simulink model "UART"  (R2025a)
settings: Solver=FixedStepAuto  StartTime=0.0  StopTime=10  FixedStep=1e-6  RelTol=1e-3
undefined symbols (not defined in the file): Bit_1, Bit_2, Bit_3, Bit_4, Bit_5, Bit_6, Bit_7, Bit_8
libraries: simulink_extras x158, fl_lib x17, nesl_utility x8, simulink x7
(part 3 of 6)

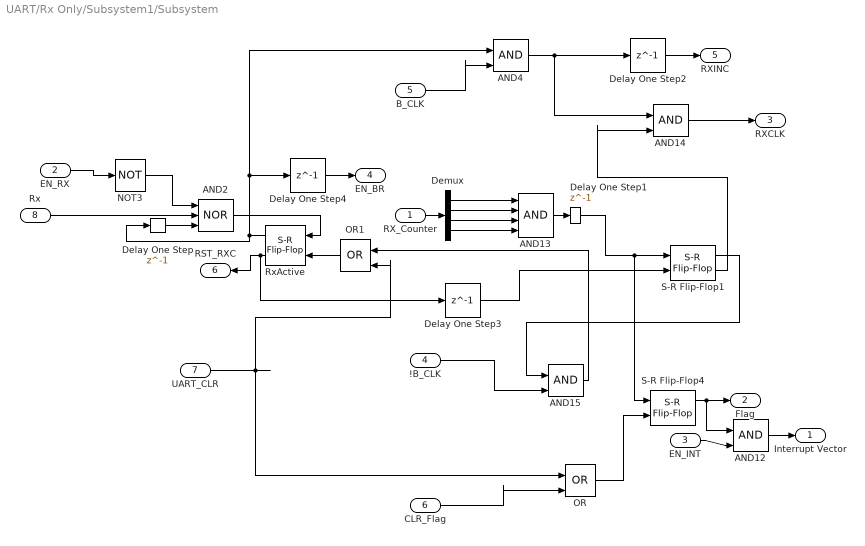
== system UART/Rx Only/Subsystem1/Subsystem ==
  RX_Counter : Inport
  EN_RX : Inport  Port=2
  EN_INT : Inport  Port=3
  !B_CLK : Inport  Port=4
  B_CLK : Inport  Port=5
  CLR_Flag : Inport  Port=6
  UART_CLR : Inport  Port=7
  Rx : Inport  Port=8
  AND{4,12,14..15} (4 alike) : Logic  IconShape=distinctive  AllPortsSameDT=off  OutDataTypeStr=boolean
  AND13 : Logic  Inputs=4  IconShape=distinctive  AllPortsSameDT=off  OutDataTypeStr=boolean
  AND2 : Logic  Operator=NOR  Inputs=3  IconShape=distinctive  AllPortsSameDT=off  OutDataTypeStr=boolean
  Delay One Step{,1..4} (5 alike) : Delay  DelayLength=1
  Demux : Demux
  NOT3 : Logic  Operator=NOT  IconShape=distinctive  AllPortsSameDT=off  OutDataTypeStr=boolean
  OR : Logic  Operator=OR  IconShape=distinctive  AllPortsSameDT=off  OutDataTypeStr=boolean
  OR1 : Logic  Operator=OR  IconShape=distinctive  AllPortsSameDT=off  OutDataTypeStr=boolean
  RxActive : simulink_extras/Flip Flops/S-R Flip-Flop  initial_condition=0
  S-R Flip-Flop1 : simulink_extras/Flip Flops/S-R Flip-Flop  initial_condition=0
  S-R Flip-Flop4 : simulink_extras/Flip Flops/S-R Flip-Flop  initial_condition=0
  Interrupt Vector : Outport
  Flag : Outport  Port=2
  RXCLK : Outport  Port=3
  EN_BR : Outport  Port=4
  RXINC : Outport  Port=5
  RST_RXC : Outport  Port=6
  wires:
  UART_CLR/1 -> OR/1, OR1/2
  !B_CLK/1 -> AND15/2
  Rx/1 -> AND2/2
  EN_RX/1 -> NOT3/1
  AND2/1 -> RxActive/1
  EN_INT/1 -> AND12/2
  S-R Flip-Flop4/1 -> AND12/1, Flag/1
  AND12/1 -> Interrupt Vector/1
  CLR_Flag/1 -> OR/2
  RxActive/2 -> Delay One Step3/1, RST_RXC/1
  Demux/1 -> AND13/1
  Demux/2 -> AND13/2
  B_CLK/1 -> AND4/2
  AND4/1 -> Delay One Step2/1, AND14/1
  RX_Counter/1 -> Demux/1
  Delay One Step1/1 -> S-R Flip-Flop4/1, S-R Flip-Flop1/1
  AND15/1 -> OR1/1
  RxActive/1 -> Delay One Step/1, Delay One Step4/1, AND4/1
  Demux/3 -> AND13/3
  Demux/4 -> AND13/4
  Delay One Step2/1 -> RXINC/1
  AND14/1 -> RXCLK/1
  S-R Flip-Flop1/2 -> AND14/2
  OR1/1 -> RxActive/2
  NOT3/1 -> AND2/1
  Delay One Step/1 -> AND2/3
  AND13/1 -> Delay One Step1/1
  OR/1 -> S-R Flip-Flop4/2
  S-R Flip-Flop1/1 -> AND15/1
  Delay One Step3/1 -> S-R Flip-Flop1/2
  Delay One Step4/1 -> EN_BR/1

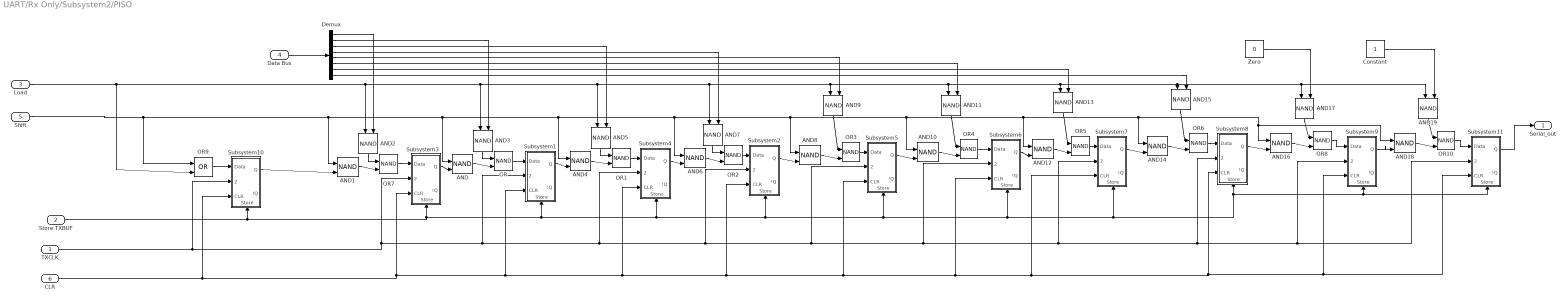
== system UART/Rx Only/Subsystem2/PISO ==
  "TXCLK " : Inport
  Store TXBUF : Inport  Port=2
  Load : Inport  Port=3
  Data Bus : Inport  Port=4
  Shift : Inport  Port=5
  "CLR " : Inport  Port=6
  AND{,1..19} (20 alike) : Logic  Operator=NAND  IconShape=distinctive  AllPortsSameDT=off  OutDataTypeStr=boolean
  Constant : Constant
  Demux : Demux  Outputs=8
  OR{,1..8,10} (10 alike) : Logic  Operator=NAND  IconShape=distinctive  AllPortsSameDT=off  OutDataTypeStr=boolean
  OR9 : Logic  Operator=OR  IconShape=distinctive  AllPortsSameDT=off  OutDataTypeStr=boolean
  Subsystem1 : Subsystem
      settings: PortSchema="{\"entries\":[{\"content\":{\"sides\":[{\"content\":{\"connectorIds\":[\"In1\",\"In2\",\"In3\"]},\"type\":\"ConnectorPlacement.EquallySpacedRectSide\",\"uuid\":\"7f3c85a8-435a-48c3-b59c-f5d5714c847e\"},{\"content\":{\"connectorIds\":[\"Out1\",\"Out2\"],\"side\":\"RIGHT\"},\"type\":\"ConnectorPlacement.EquallySpacedRectSide\",\"uuid\":\"17207f13-8340-45d6-91b4-1610668ce323\"},{\"content\":{\"side\":\"TOP\"},\"type\":\"ConnectorPlacement.EquallySpacedRectSide\",\"uuid\":\"04d61695-a4c9-4852-a4b1-2cdbdbfa921f\"},{\"content\":{\"connectorIds\":[\"In4\"],\"side\":\"BOTTOM\"},\"type\":\"ConnectorPlacement.EquallySpacedRectSide\",\"uuid\":\"a1770489-59eb-478b-9b54-00148a18765c\"}]},\"type\":\"ConnectorPlacement.EquallySpacedConnector\",\"uuid\":\"06dc9f9c-9f45-42f3-b967-f8303bc685fc\"}],\"packageUris\":[\"http://schema.mathworks.com/mf0/Connector/R2020b\"],\"version\":\"1.0\"}"
  Subsystem10 : Subsystem
      settings: PortSchema="{\"entries\":[{\"content\":{\"sides\":[{\"content\":{\"connectorIds\":[\"In1\",\"In2\",\"In3\"]},\"type\":\"ConnectorPlacement.EquallySpacedRectSide\",\"uuid\":\"7f3c85a8-435a-48c3-b59c-f5d5714c847e\"},{\"content\":{\"connectorIds\":[\"Out1\",\"Out2\"],\"side\":\"RIGHT\"},\"type\":\"ConnectorPlacement.EquallySpacedRectSide\",\"uuid\":\"17207f13-8340-45d6-91b4-1610668ce323\"},{\"content\":{\"side\":\"TOP\"},\"type\":\"ConnectorPlacement.EquallySpacedRectSide\",\"uuid\":\"04d61695-a4c9-4852-a4b1-2cdbdbfa921f\"},{\"content\":{\"connectorIds\":[\"In4\"],\"side\":\"BOTTOM\"},\"type\":\"ConnectorPlacement.EquallySpacedRectSide\",\"uuid\":\"a1770489-59eb-478b-9b54-00148a18765c\"}]},\"type\":\"ConnectorPlacement.EquallySpacedConnector\",\"uuid\":\"06dc9f9c-9f45-42f3-b967-f8303bc685fc\"}],\"packageUris\":[\"http://schema.mathworks.com/mf0/Connector/R2020b\"],\"version\":\"1.0\"}"
  Subsystem11 : Subsystem
      settings: PortSchema="{\"entries\":[{\"content\":{\"sides\":[{\"content\":{\"connectorIds\":[\"In1\",\"In2\",\"In3\"]},\"type\":\"ConnectorPlacement.EquallySpacedRectSide\",\"uuid\":\"7f3c85a8-435a-48c3-b59c-f5d5714c847e\"},{\"content\":{\"connectorIds\":[\"Out1\",\"Out2\"],\"side\":\"RIGHT\"},\"type\":\"ConnectorPlacement.EquallySpacedRectSide\",\"uuid\":\"17207f13-8340-45d6-91b4-1610668ce323\"},{\"content\":{\"side\":\"TOP\"},\"type\":\"ConnectorPlacement.EquallySpacedRectSide\",\"uuid\":\"04d61695-a4c9-4852-a4b1-2cdbdbfa921f\"},{\"content\":{\"connectorIds\":[\"In4\"],\"side\":\"BOTTOM\"},\"type\":\"ConnectorPlacement.EquallySpacedRectSide\",\"uuid\":\"a1770489-59eb-478b-9b54-00148a18765c\"}]},\"type\":\"ConnectorPlacement.EquallySpacedConnector\",\"uuid\":\"06dc9f9c-9f45-42f3-b967-f8303bc685fc\"}],\"packageUris\":[\"http://schema.mathworks.com/mf0/Connector/R2020b\"],\"version\":\"1.0\"}"
  Subsystem2 : Subsystem
      settings: PortSchema="{\"entries\":[{\"content\":{\"sides\":[{\"content\":{\"connectorIds\":[\"In1\",\"In2\",\"In3\"]},\"type\":\"ConnectorPlacement.EquallySpacedRectSide\",\"uuid\":\"7f3c85a8-435a-48c3-b59c-f5d5714c847e\"},{\"content\":{\"connectorIds\":[\"Out1\",\"Out2\"],\"side\":\"RIGHT\"},\"type\":\"ConnectorPlacement.EquallySpacedRectSide\",\"uuid\":\"17207f13-8340-45d6-91b4-1610668ce323\"},{\"content\":{\"side\":\"TOP\"},\"type\":\"ConnectorPlacement.EquallySpacedRectSide\",\"uuid\":\"04d61695-a4c9-4852-a4b1-2cdbdbfa921f\"},{\"content\":{\"connectorIds\":[\"In4\"],\"side\":\"BOTTOM\"},\"type\":\"ConnectorPlacement.EquallySpacedRectSide\",\"uuid\":\"a1770489-59eb-478b-9b54-00148a18765c\"}]},\"type\":\"ConnectorPlacement.EquallySpacedConnector\",\"uuid\":\"06dc9f9c-9f45-42f3-b967-f8303bc685fc\"}],\"packageUris\":[\"http://schema.mathworks.com/mf0/Connector/R2020b\"],\"version\":\"1.0\"}"
  Subsystem3 : Subsystem
      settings: PortSchema="{\"entries\":[{\"content\":{\"sides\":[{\"content\":{\"connectorIds\":[\"In1\",\"In2\",\"In3\"]},\"type\":\"ConnectorPlacement.EquallySpacedRectSide\",\"uuid\":\"7f3c85a8-435a-48c3-b59c-f5d5714c847e\"},{\"content\":{\"connectorIds\":[\"Out1\",\"Out2\"],\"side\":\"RIGHT\"},\"type\":\"ConnectorPlacement.EquallySpacedRectSide\",\"uuid\":\"17207f13-8340-45d6-91b4-1610668ce323\"},{\"content\":{\"side\":\"TOP\"},\"type\":\"ConnectorPlacement.EquallySpacedRectSide\",\"uuid\":\"04d61695-a4c9-4852-a4b1-2cdbdbfa921f\"},{\"content\":{\"connectorIds\":[\"In4\"],\"side\":\"BOTTOM\"},\"type\":\"ConnectorPlacement.EquallySpacedRectSide\",\"uuid\":\"a1770489-59eb-478b-9b54-00148a18765c\"}]},\"type\":\"ConnectorPlacement.EquallySpacedConnector\",\"uuid\":\"06dc9f9c-9f45-42f3-b967-f8303bc685fc\"}],\"packageUris\":[\"http://schema.mathworks.com/mf0/Connector/R2020b\"],\"version\":\"1.0\"}"
  Subsystem4 : Subsystem
      settings: PortSchema="{\"entries\":[{\"content\":{\"sides\":[{\"content\":{\"connectorIds\":[\"In1\",\"In2\",\"In3\"]},\"type\":\"ConnectorPlacement.EquallySpacedRectSide\",\"uuid\":\"7f3c85a8-435a-48c3-b59c-f5d5714c847e\"},{\"content\":{\"connectorIds\":[\"Out1\",\"Out2\"],\"side\":\"RIGHT\"},\"type\":\"ConnectorPlacement.EquallySpacedRectSide\",\"uuid\":\"17207f13-8340-45d6-91b4-1610668ce323\"},{\"content\":{\"side\":\"TOP\"},\"type\":\"ConnectorPlacement.EquallySpacedRectSide\",\"uuid\":\"04d61695-a4c9-4852-a4b1-2cdbdbfa921f\"},{\"content\":{\"connectorIds\":[\"In4\"],\"side\":\"BOTTOM\"},\"type\":\"ConnectorPlacement.EquallySpacedRectSide\",\"uuid\":\"a1770489-59eb-478b-9b54-00148a18765c\"}]},\"type\":\"ConnectorPlacement.EquallySpacedConnector\",\"uuid\":\"06dc9f9c-9f45-42f3-b967-f8303bc685fc\"}],\"packageUris\":[\"http://schema.mathworks.com/mf0/Connector/R2020b\"],\"version\":\"1.0\"}"
  Subsystem5 : Subsystem
      settings: PortSchema="{\"entries\":[{\"content\":{\"sides\":[{\"content\":{\"connectorIds\":[\"In1\",\"In2\",\"In3\"]},\"type\":\"ConnectorPlacement.EquallySpacedRectSide\",\"uuid\":\"7f3c85a8-435a-48c3-b59c-f5d5714c847e\"},{\"content\":{\"connectorIds\":[\"Out1\",\"Out2\"],\"side\":\"RIGHT\"},\"type\":\"ConnectorPlacement.EquallySpacedRectSide\",\"uuid\":\"17207f13-8340-45d6-91b4-1610668ce323\"},{\"content\":{\"side\":\"TOP\"},\"type\":\"ConnectorPlacement.EquallySpacedRectSide\",\"uuid\":\"04d61695-a4c9-4852-a4b1-2cdbdbfa921f\"},{\"content\":{\"connectorIds\":[\"In4\"],\"side\":\"BOTTOM\"},\"type\":\"ConnectorPlacement.EquallySpacedRectSide\",\"uuid\":\"a1770489-59eb-478b-9b54-00148a18765c\"}]},\"type\":\"ConnectorPlacement.EquallySpacedConnector\",\"uuid\":\"06dc9f9c-9f45-42f3-b967-f8303bc685fc\"}],\"packageUris\":[\"http://schema.mathworks.com/mf0/Connector/R2020b\"],\"version\":\"1.0\"}"
  Subsystem6 : Subsystem
      settings: PortSchema="{\"entries\":[{\"content\":{\"sides\":[{\"content\":{\"connectorIds\":[\"In1\",\"In2\",\"In3\"]},\"type\":\"ConnectorPlacement.EquallySpacedRectSide\",\"uuid\":\"7f3c85a8-435a-48c3-b59c-f5d5714c847e\"},{\"content\":{\"connectorIds\":[\"Out1\",\"Out2\"],\"side\":\"RIGHT\"},\"type\":\"ConnectorPlacement.EquallySpacedRectSide\",\"uuid\":\"17207f13-8340-45d6-91b4-1610668ce323\"},{\"content\":{\"side\":\"TOP\"},\"type\":\"ConnectorPlacement.EquallySpacedRectSide\",\"uuid\":\"04d61695-a4c9-4852-a4b1-2cdbdbfa921f\"},{\"content\":{\"connectorIds\":[\"In4\"],\"side\":\"BOTTOM\"},\"type\":\"ConnectorPlacement.EquallySpacedRectSide\",\"uuid\":\"a1770489-59eb-478b-9b54-00148a18765c\"}]},\"type\":\"ConnectorPlacement.EquallySpacedConnector\",\"uuid\":\"06dc9f9c-9f45-42f3-b967-f8303bc685fc\"}],\"packageUris\":[\"http://schema.mathworks.com/mf0/Connector/R2020b\"],\"version\":\"1.0\"}"
  Subsystem7 : Subsystem
      settings: PortSchema="{\"entries\":[{\"content\":{\"sides\":[{\"content\":{\"connectorIds\":[\"In1\",\"In2\",\"In3\"]},\"type\":\"ConnectorPlacement.EquallySpacedRectSide\",\"uuid\":\"7f3c85a8-435a-48c3-b59c-f5d5714c847e\"},{\"content\":{\"connectorIds\":[\"Out1\",\"Out2\"],\"side\":\"RIGHT\"},\"type\":\"ConnectorPlacement.EquallySpacedRectSide\",\"uuid\":\"17207f13-8340-45d6-91b4-1610668ce323\"},{\"content\":{\"side\":\"TOP\"},\"type\":\"ConnectorPlacement.EquallySpacedRectSide\",\"uuid\":\"04d61695-a4c9-4852-a4b1-2cdbdbfa921f\"},{\"content\":{\"connectorIds\":[\"In4\"],\"side\":\"BOTTOM\"},\"type\":\"ConnectorPlacement.EquallySpacedRectSide\",\"uuid\":\"a1770489-59eb-478b-9b54-00148a18765c\"}]},\"type\":\"ConnectorPlacement.EquallySpacedConnector\",\"uuid\":\"06dc9f9c-9f45-42f3-b967-f8303bc685fc\"}],\"packageUris\":[\"http://schema.mathworks.com/mf0/Connector/R2020b\"],\"version\":\"1.0\"}"
  Subsystem8 : Subsystem
      settings: PortSchema="{\"entries\":[{\"content\":{\"sides\":[{\"content\":{\"connectorIds\":[\"In1\",\"In2\",\"In3\"]},\"type\":\"ConnectorPlacement.EquallySpacedRectSide\",\"uuid\":\"7f3c85a8-435a-48c3-b59c-f5d5714c847e\"},{\"content\":{\"connectorIds\":[\"Out1\",\"Out2\"],\"side\":\"RIGHT\"},\"type\":\"ConnectorPlacement.EquallySpacedRectSide\",\"uuid\":\"17207f13-8340-45d6-91b4-1610668ce323\"},{\"content\":{\"side\":\"TOP\"},\"type\":\"ConnectorPlacement.EquallySpacedRectSide\",\"uuid\":\"04d61695-a4c9-4852-a4b1-2cdbdbfa921f\"},{\"content\":{\"connectorIds\":[\"In4\"],\"side\":\"BOTTOM\"},\"type\":\"ConnectorPlacement.EquallySpacedRectSide\",\"uuid\":\"a1770489-59eb-478b-9b54-00148a18765c\"}]},\"type\":\"ConnectorPlacement.EquallySpacedConnector\",\"uuid\":\"06dc9f9c-9f45-42f3-b967-f8303bc685fc\"}],\"packageUris\":[\"http://schema.mathworks.com/mf0/Connector/R2020b\"],\"version\":\"1.0\"}"
  Subsystem9 : Subsystem
      settings: PortSchema="{\"entries\":[{\"content\":{\"sides\":[{\"content\":{\"connectorIds\":[\"In1\",\"In2\",\"In3\"]},\"type\":\"ConnectorPlacement.EquallySpacedRectSide\",\"uuid\":\"7f3c85a8-435a-48c3-b59c-f5d5714c847e\"},{\"content\":{\"connectorIds\":[\"Out1\",\"Out2\"],\"side\":\"RIGHT\"},\"type\":\"ConnectorPlacement.EquallySpacedRectSide\",\"uuid\":\"17207f13-8340-45d6-91b4-1610668ce323\"},{\"content\":{\"side\":\"TOP\"},\"type\":\"ConnectorPlacement.EquallySpacedRectSide\",\"uuid\":\"04d61695-a4c9-4852-a4b1-2cdbdbfa921f\"},{\"content\":{\"connectorIds\":[\"In4\"],\"side\":\"BOTTOM\"},\"type\":\"ConnectorPlacement.EquallySpacedRectSide\",\"uuid\":\"a1770489-59eb-478b-9b54-00148a18765c\"}]},\"type\":\"ConnectorPlacement.EquallySpacedConnector\",\"uuid\":\"06dc9f9c-9f45-42f3-b967-f8303bc685fc\"}],\"packageUris\":[\"http://schema.mathworks.com/mf0/Connector/R2020b\"],\"version\":\"1.0\"}"
  Zero : Constant  Value=0  OutDataTypeStr=Inherit: Inherit via back propagation
  Serial_out : Outport
  wires:
  AND12/1 -> OR5/2
  AND14/1 -> OR6/2
  AND13/1 -> OR5/1
  OR6/1 -> Subsystem8/1(Data)
  AND6/1 -> OR2/2
  AND7/1 -> OR2/1
  Subsystem4/1(Q) -> AND6/2
  OR2/1 -> Subsystem2/1(Data)
  Subsystem2/1(Q) -> AND8/2
  AND15/1 -> OR6/1
  AND8/1 -> OR3/2
  AND3/1 -> OR/1
  OR5/1 -> Subsystem7/1(Data)
  Subsystem7/1(Q) -> AND14/2
  AND11/1 -> OR4/1
  AND9/1 -> OR3/1
  Subsystem6/1(Q) -> AND12/2
  OR3/1 -> Subsystem5/1(Data)
  OR4/1 -> Subsystem6/1(Data)
  OR1/1 -> Subsystem4/1(Data)
  AND5/1 -> OR1/1
  AND/1 -> OR/2
  AND4/1 -> OR1/2
  Subsystem1/1(Q) -> AND4/2
  Subsystem3/1(Q) -> AND/2
  OR/1 -> Subsystem1/1(Data)
  OR7/1 -> Subsystem3/1(Data)
  Subsystem5/1(Q) -> AND10/2
  AND10/1 -> OR4/2
  Data Bus/1 -> Demux/1
  AND2/1 -> OR7/1
  AND1/1 -> OR7/2
  Subsystem8/1(Q) -> AND16/2
  Subsystem10/1(Q) -> AND1/2
  Demux/1 -> AND2/2
  Demux/2 -> AND3/2
  Demux/3 -> AND5/2
  Demux/4 -> AND7/2
  Demux/5 -> AND9/2
  Demux/6 -> AND11/2
  Demux/7 -> AND13/2
  Demux/8 -> AND15/2
  AND16/1 -> OR8/2
  OR8/1 -> Subsystem9/1(Data)
  AND17/1 -> OR8/1
  Zero/1 -> AND17/2
  OR9/1 -> Subsystem10/1(Data)
  Subsystem11/1(Q) -> Serial_out/1
  Load/1 -> OR9/2, AND2/1, AND3/1, AND5/1, AND7/1, AND9/1, AND11/1, AND13/1, AND19/1, AND17/1, AND15/1
  OR10/1 -> Subsystem11/1(Data)
  "TXCLK "/1 -> Subsystem10/2(Clock), Subsystem3/2(Clock), Subsystem1/2(Clock), Subsystem4/2(Clock), Subsystem2/2(Clock), Subsystem5/2(Clock), Subsystem6/2(Clock), Subsystem11/2(Clock), Subsystem9/2(Clock), Subsystem8/2(Clock), Subsystem7/2(Clock)
  Subsystem9/1(Q) -> AND18/2
  AND19/1 -> OR10/1
  AND18/1 -> OR10/2
  Store TXBUF/1 -> Subsystem10/4(Store), Subsystem3/4(Store), Subsystem1/4(Store), Subsystem4/4(Store), Subsystem2/4(Store), Subsystem5/4(Store), Subsystem6/4(Store), Subsystem11/4(Store), Subsystem9/4(Store), Subsystem8/4(Store), Subsystem7/4(Store)
  Constant/1 -> AND19/2
  "CLR "/1 -> Subsystem10/3(CLR), Subsystem3/3(CLR), Subsystem1/3(CLR), Subsystem4/3(CLR), Subsystem2/3(CLR), Subsystem5/3(CLR), Subsystem6/3(CLR), Subsystem11/3(CLR), Subsystem9/3(CLR), Subsystem8/3(CLR), Subsystem7/3(CLR)
  Shift/1 -> OR9/1, AND1/1, AND6/1, AND10/1, AND12/1, AND18/1, AND16/1, AND14/1, AND8/1, AND4/1, AND/1

== system UART/Rx Only/Subsystem2/RX Counter1 ==
  BC_Reset : Inport
  INC : Inport  Port=2
  Constant : Constant
  D Flip-Flop{5..7,11} (4 alike) : simulink_extras/Flip Flops/D Flip-Flop
  Delay One Step : Delay  DelayLength=1
  Demux : Demux
  Half Adder : Subsystem
      settings: PortSchema="{\"entries\":[{\"content\":{\"sides\":[{\"content\":{\"connectorIds\":[\"In1\"]},\"type\":\"ConnectorPlacement.EquallySpacedRectSide\",\"uuid\":\"d3a7e232-15f2-47a9-a065-9480c81dc57e\"},{\"content\":{\"connectorIds\":[\"Out1\"],\"side\":\"RIGHT\"},\"type\":\"ConnectorPlacement.EquallySpacedRectSide\",\"uuid\":\"e118f150-fee7-4aeb-941e-53c3f02c6791\"},{\"content\":{\"connectorIds\":[\"Out2\"],\"side\":\"TOP\"},\"type\":\"ConnectorPlacement.EquallySpacedRectSide\",\"uuid\":\"6d9038ab-faad-455b-a9c5-8fe0bbf34e51\"},{\"content\":{\"connectorIds\":[\"In2\"],\"side\":\"BOTTOM\"},\"type\":\"ConnectorPlacement.EquallySpacedRectSide\",\"uuid\":\"d09c8d4f-08f3-4c52-88a6-8c6db517fc7a\"}]},\"type\":\"ConnectorPlacement.EquallySpacedConnector\",\"uuid\":\"5bc947ce-f1cd-4957-9186-40c14c78de7d\"}],\"packageUris\":[\"http://schema.mathworks.com/mf0/Connector/R2020b\"],\"version\":\"1.0\"}"
  Half Adder1 : Subsystem
      settings: PortSchema="{\"entries\":[{\"content\":{\"sides\":[{\"content\":{\"connectorIds\":[\"In1\"]},\"type\":\"ConnectorPlacement.EquallySpacedRectSide\",\"uuid\":\"d3a7e232-15f2-47a9-a065-9480c81dc57e\"},{\"content\":{\"connectorIds\":[\"Out1\"],\"side\":\"RIGHT\"},\"type\":\"ConnectorPlacement.EquallySpacedRectSide\",\"uuid\":\"e118f150-fee7-4aeb-941e-53c3f02c6791\"},{\"content\":{\"connectorIds\":[\"Out2\"],\"side\":\"TOP\"},\"type\":\"ConnectorPlacement.EquallySpacedRectSide\",\"uuid\":\"6d9038ab-faad-455b-a9c5-8fe0bbf34e51\"},{\"content\":{\"connectorIds\":[\"In2\"],\"side\":\"BOTTOM\"},\"type\":\"ConnectorPlacement.EquallySpacedRectSide\",\"uuid\":\"d09c8d4f-08f3-4c52-88a6-8c6db517fc7a\"}]},\"type\":\"ConnectorPlacement.EquallySpacedConnector\",\"uuid\":\"5bc947ce-f1cd-4957-9186-40c14c78de7d\"}],\"packageUris\":[\"http://schema.mathworks.com/mf0/Connector/R2020b\"],\"version\":\"1.0\"}"
  Half Adder2 : Subsystem
      settings: PortSchema="{\"entries\":[{\"content\":{\"sides\":[{\"content\":{\"connectorIds\":[\"In1\"]},\"type\":\"ConnectorPlacement.EquallySpacedRectSide\",\"uuid\":\"d3a7e232-15f2-47a9-a065-9480c81dc57e\"},{\"content\":{\"connectorIds\":[\"Out1\"],\"side\":\"RIGHT\"},\"type\":\"ConnectorPlacement.EquallySpacedRectSide\",\"uuid\":\"e118f150-fee7-4aeb-941e-53c3f02c6791\"},{\"content\":{\"connectorIds\":[\"Out2\"],\"side\":\"TOP\"},\"type\":\"ConnectorPlacement.EquallySpacedRectSide\",\"uuid\":\"6d9038ab-faad-455b-a9c5-8fe0bbf34e51\"},{\"content\":{\"connectorIds\":[\"In2\"],\"side\":\"BOTTOM\"},\"type\":\"ConnectorPlacement.EquallySpacedRectSide\",\"uuid\":\"d09c8d4f-08f3-4c52-88a6-8c6db517fc7a\"}]},\"type\":\"ConnectorPlacement.EquallySpacedConnector\",\"uuid\":\"5bc947ce-f1cd-4957-9186-40c14c78de7d\"}],\"packageUris\":[\"http://schema.mathworks.com/mf0/Connector/R2020b\"],\"version\":\"1.0\"}"
  Half Adder7 : Subsystem
      settings: PortSchema="{\"entries\":[{\"content\":{\"sides\":[{\"content\":{\"connectorIds\":[\"In1\"]},\"type\":\"ConnectorPlacement.EquallySpacedRectSide\",\"uuid\":\"d3a7e232-15f2-47a9-a065-9480c81dc57e\"},{\"content\":{\"connectorIds\":[\"Out1\"],\"side\":\"RIGHT\"},\"type\":\"ConnectorPlacement.EquallySpacedRectSide\",\"uuid\":\"e118f150-fee7-4aeb-941e-53c3f02c6791\"},{\"content\":{\"connectorIds\":[\"Out2\"],\"side\":\"TOP\"},\"type\":\"ConnectorPlacement.EquallySpacedRectSide\",\"uuid\":\"6d9038ab-faad-455b-a9c5-8fe0bbf34e51\"},{\"content\":{\"connectorIds\":[\"In2\"],\"side\":\"BOTTOM\"},\"type\":\"ConnectorPlacement.EquallySpacedRectSide\",\"uuid\":\"d09c8d4f-08f3-4c52-88a6-8c6db517fc7a\"}]},\"type\":\"ConnectorPlacement.EquallySpacedConnector\",\"uuid\":\"5bc947ce-f1cd-4957-9186-40c14c78de7d\"}],\"packageUris\":[\"http://schema.mathworks.com/mf0/Connector/R2020b\"],\"version\":\"1.0\"}"
  Mux1 : Mux
  NOT : Logic  Operator=NOT  IconShape=distinctive  AllPortsSameDT=off  OutDataTypeStr=boolean
  C4 : Outport
  !C3 : Outport  Port=2
  C2 : Outport  Port=3
  C1 : Outport  Port=4
  wires:
  Mux1/1 -> Delay One Step/1
  BC_Reset/1 -> NOT/1
  Delay One Step/1 -> Demux/1
  Demux/4 -> D Flip-Flop7/1
  Demux/3 -> D Flip-Flop5/1
  Demux/2 -> D Flip-Flop6/1
  Demux/1 -> D Flip-Flop11/1
  INC/1 -> D Flip-Flop11/2, D Flip-Flop6/2, D Flip-Flop5/2, D Flip-Flop7/2
  Constant/1 -> Half Adder7/2("B ")
  Half Adder/2(Carry) -> Half Adder1/2("B ")
  Half Adder1/1(Sum) -> Mux1/2
  Half Adder/1(Sum) -> Mux1/3
  Half Adder2/1(Sum) -> Mux1/1
  Half Adder1/2(Carry) -> Half Adder2/2("B ")
  Half Adder7/1(Sum) -> Mux1/4
  Half Adder7/2(Carry) -> Half Adder/2("B ")
  D Flip-Flop11/1 -> C4/1, Half Adder2/1(A)  "D1"
  D Flip-Flop6/1 -> Half Adder1/1(A)  "D3"
  D Flip-Flop5/1 -> C2/1, Half Adder/1(A)  "D4"
  D Flip-Flop7/1 -> C1/1, Half Adder7/1(A)  "D2"
  NOT/1 -> D Flip-Flop11/3, D Flip-Flop6/3, D Flip-Flop5/3, D Flip-Flop7/3
  D Flip-Flop6/2 -> !C3/1

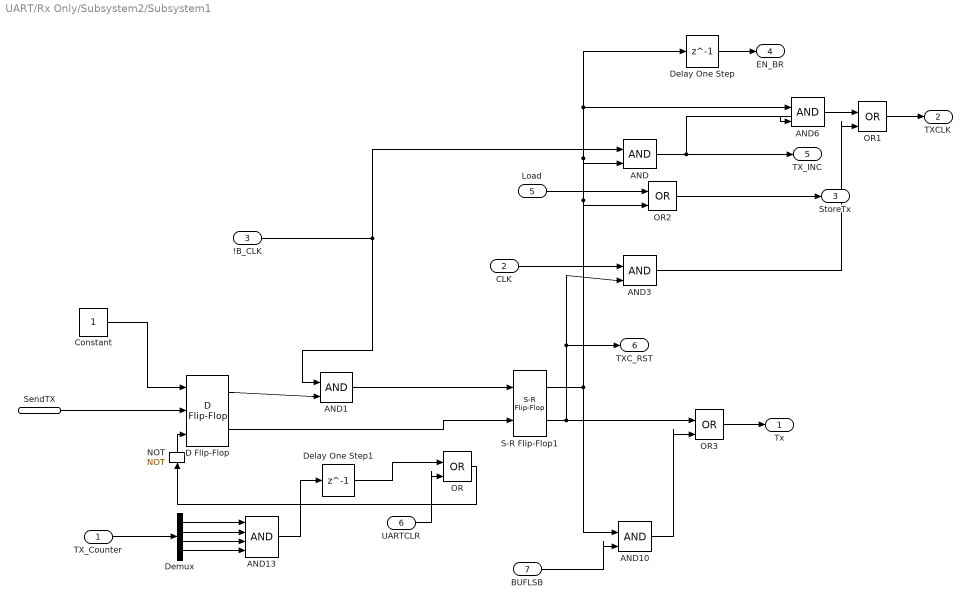
== system UART/Rx Only/Subsystem2/Subsystem1 ==
  TX_Counter : Inport
  CLK : Inport  Port=2
  !B_CLK : Inport  Port=3
  SendTX : Inport  Port=4
  Load : Inport  Port=5
  UARTCLR : Inport  Port=6
  BUFLSB : Inport  Port=7
  AND{,1,3,6,10} (5 alike) : Logic  IconShape=distinctive  AllPortsSameDT=off  OutDataTypeStr=boolean
  AND13 : Logic  Inputs=4  IconShape=distinctive  AllPortsSameDT=off  OutDataTypeStr=boolean
  Constant : Constant  OutDataTypeStr=boolean
  D Flip-Flop : simulink_extras/Flip Flops/D Flip-Flop
  Delay One Step : Delay  DelayLength=1
  Delay One Step1 : Delay  DelayLength=1  SampleTime=1e-5
  Demux : Demux
  NOT : Logic  Operator=NOT  IconShape=distinctive  AllPortsSameDT=off  OutDataTypeStr=boolean
  OR{,1..3} (4 alike) : Logic  Operator=OR  IconShape=distinctive  AllPortsSameDT=off  OutDataTypeStr=boolean
  S-R Flip-Flop1 : simulink_extras/Flip Flops/S-R Flip-Flop  initial_condition=0
  Tx : Outport
  TXCLK : Outport  Port=2
  StoreTx : Outport  Port=3
  EN_BR : Outport  Port=4
  TX_INC : Outport  Port=5
  TXC_RST : Outport  Port=6
  wires:
  OR2/1 -> StoreTx/1
  AND3/1 -> OR1/2
  S-R Flip-Flop1/2 -> AND3/2, TXC_RST/1, OR3/1
  CLK/1 -> AND3/1
  OR1/1 -> TXCLK/1
  SendTX/1 -> D Flip-Flop/2
  Delay One Step1/1 -> OR/1
  S-R Flip-Flop1/1 -> AND10/1, AND6/1, Delay One Step/1, AND/2, OR2/2
  Load/1 -> OR2/1
  BUFLSB/1 -> AND10/2
  AND/1 -> AND6/2, TX_INC/1
  AND10/1 -> OR3/2
  AND6/1 -> OR1/1
  OR3/1 -> Tx/1
  TX_Counter/1 -> Demux/1
  Delay One Step/1 -> EN_BR/1
  Demux/1 -> AND13/1
  Demux/2 -> AND13/2
  Demux/4 -> AND13/4
  AND13/1 -> Delay One Step1/1
  Demux/3 -> AND13/3
  !B_CLK/1 -> AND/1, AND1/1
  D Flip-Flop/1 -> AND1/2
  AND1/1 -> S-R Flip-Flop1/1
  UARTCLR/1 -> OR/2
  Constant/1 -> D Flip-Flop/1
  OR/1 -> NOT/1
  NOT/1 -> D Flip-Flop/3
  D Flip-Flop/2 -> S-R Flip-Flop1/2

== system UART/Subsystem1/Baudrate Generator/BPS ==
  Data bus : Inport
  Store : Inport  Port=2
  CLK : Inport  Port=3
  CLR : Inport  Port=4
  Demux : Demux  Outputs=8
  Mux : Mux  Inputs=8
  Subsystem1 : Subsystem
  Subsystem2 : Subsystem
  Subsystem3 : Subsystem
  Subsystem4 : Subsystem
  Subsystem5 : Subsystem
  Subsystem6 : Subsystem
  Subsystem7 : Subsystem
  Subsystem8 : Subsystem
  "Q Bus " : Outport
  wires:
  Demux/4 -> Subsystem2/1(Data)
  Mux/1 -> "Q Bus "/1
  Demux/2 -> Subsystem1/1(Data)
  Data bus/1 -> Demux/1
  Subsystem6/1(Q) -> Mux/8
  Store/1 -> Subsystem1/2(Store), Subsystem4/2(Store), Subsystem2/2(Store), Subsystem7/2(Store), Subsystem5/2(Store), Subsystem6/2(Store), Subsystem8/2(Store), Subsystem3/2(Store)
  Demux/5 -> Subsystem7/1(Data)
  Demux/7 -> Subsystem8/1(Data)
  Demux/3 -> Subsystem4/1(Data)
  Subsystem7/1(Q) -> Mux/5
  Demux/6 -> Subsystem5/1(Data)
  Subsystem1/1(Q) -> Mux/2
  Demux/1 -> Subsystem3/1(Data)
  Subsystem3/1(Q) -> Mux/1
  Demux/8 -> Subsystem6/1(Data)
  Subsystem8/1(Q) -> Mux/7
  Subsystem2/1(Q) -> Mux/4
  Subsystem4/1(Q) -> Mux/3
  Subsystem5/1(Q) -> Mux/6
  CLK/1 -> Subsystem1/3(Clock), Subsystem4/3(Clock), Subsystem2/3(Clock), Subsystem7/3(Clock), Subsystem5/3(Clock), Subsystem6/3(Clock), Subsystem8/3(Clock), Subsystem3/3(Clock)
  CLR/1 -> Subsystem8/4(Clear), Subsystem5/4(Clear), Subsystem7/4(Clear), Subsystem2/4(Clear), Subsystem4/4(Clear), Subsystem1/4(Clear), Subsystem3/4(Clear), Subsystem6/4(Clear)

== system UART/Subsystem1/Baudrate Generator/BR ==
  Data bus : Inport
  Store : Inport  Port=2
  CLK : Inport  Port=3
  CLR : Inport  Port=4
  Demux : Demux  Outputs=8
  Mux : Mux  Inputs=8
  Subsystem1 : Subsystem
  Subsystem2 : Subsystem
  Subsystem3 : Subsystem
  Subsystem4 : Subsystem
  Subsystem5 : Subsystem
  Subsystem6 : Subsystem
  Subsystem7 : Subsystem
  Subsystem8 : Subsystem
  "Q Bus " : Outport
  wires:
  Demux/4 -> Subsystem2/1(Data)
  Mux/1 -> "Q Bus "/1
  Demux/2 -> Subsystem1/1(Data)
  Data bus/1 -> Demux/1
  Subsystem6/1(Q) -> Mux/8
  Store/1 -> Subsystem1/2(Store), Subsystem4/2(Store), Subsystem2/2(Store), Subsystem7/2(Store), Subsystem5/2(Store), Subsystem6/2(Store), Subsystem8/2(Store), Subsystem3/2(Store)
  Demux/5 -> Subsystem7/1(Data)
  Demux/7 -> Subsystem8/1(Data)
  Demux/3 -> Subsystem4/1(Data)
  Subsystem7/1(Q) -> Mux/5
  Demux/6 -> Subsystem5/1(Data)
  Subsystem1/1(Q) -> Mux/2
  Demux/1 -> Subsystem3/1(Data)
  Subsystem3/1(Q) -> Mux/1
  Demux/8 -> Subsystem6/1(Data)
  Subsystem8/1(Q) -> Mux/7
  Subsystem2/1(Q) -> Mux/4
  Subsystem4/1(Q) -> Mux/3
  Subsystem5/1(Q) -> Mux/6
  CLK/1 -> Subsystem1/3(Clock), Subsystem4/3(Clock), Subsystem2/3(Clock), Subsystem7/3(Clock), Subsystem5/3(Clock), Subsystem6/3(Clock), Subsystem8/3(Clock), Subsystem3/3(Clock)
  CLR/1 -> Subsystem8/4(Clear), Subsystem5/4(Clear), Subsystem7/4(Clear), Subsystem2/4(Clear), Subsystem4/4(Clear), Subsystem1/4(Clear), Subsystem3/4(Clear), Subsystem6/4(Clear)

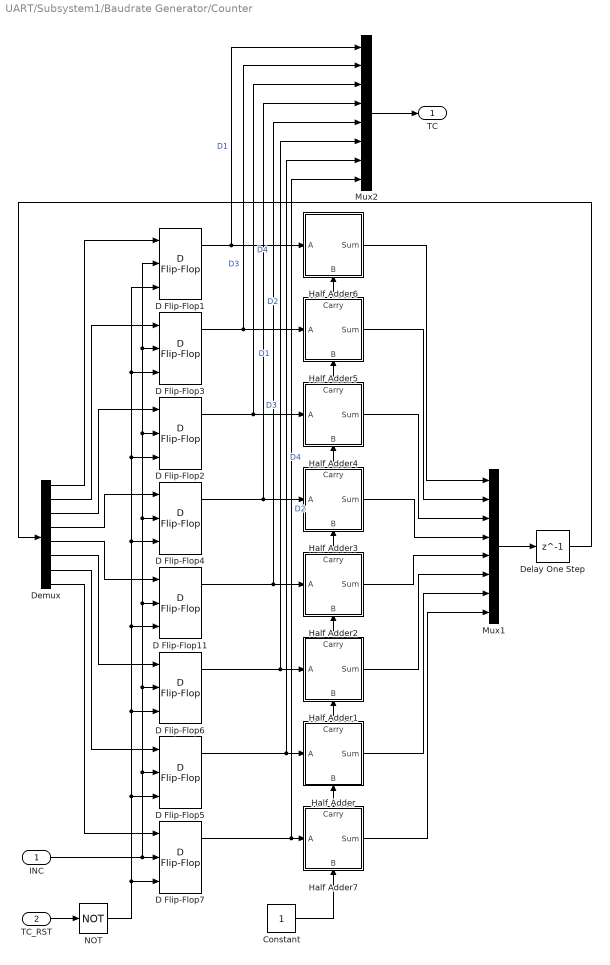
== system UART/Subsystem1/Baudrate Generator/Counter ==
  INC : Inport
  TC_RST : Inport  Port=2
  Constant : Constant
  D Flip-Flop{1..7,11} (8 alike) : simulink_extras/Flip Flops/D Flip-Flop
  Delay One Step : Delay  DelayLength=1
  Demux : Demux  Outputs=8
  Half Adder : Subsystem
      settings: PortSchema="{\"entries\":[{\"content\":{\"sides\":[{\"content\":{\"connectorIds\":[\"In1\"]},\"type\":\"ConnectorPlacement.EquallySpacedRectSide\",\"uuid\":\"d3a7e232-15f2-47a9-a065-9480c81dc57e\"},{\"content\":{\"connectorIds\":[\"Out1\"],\"side\":\"RIGHT\"},\"type\":\"ConnectorPlacement.EquallySpacedRectSide\",\"uuid\":\"e118f150-fee7-4aeb-941e-53c3f02c6791\"},{\"content\":{\"connectorIds\":[\"Out2\"],\"side\":\"TOP\"},\"type\":\"ConnectorPlacement.EquallySpacedRectSide\",\"uuid\":\"6d9038ab-faad-455b-a9c5-8fe0bbf34e51\"},{\"content\":{\"connectorIds\":[\"In2\"],\"side\":\"BOTTOM\"},\"type\":\"ConnectorPlacement.EquallySpacedRectSide\",\"uuid\":\"d09c8d4f-08f3-4c52-88a6-8c6db517fc7a\"}]},\"type\":\"ConnectorPlacement.EquallySpacedConnector\",\"uuid\":\"5bc947ce-f1cd-4957-9186-40c14c78de7d\"}],\"packageUris\":[\"http://schema.mathworks.com/mf0/Connector/R2020b\"],\"version\":\"1.0\"}"
  Half Adder1 : Subsystem
      settings: PortSchema="{\"entries\":[{\"content\":{\"sides\":[{\"content\":{\"connectorIds\":[\"In1\"]},\"type\":\"ConnectorPlacement.EquallySpacedRectSide\",\"uuid\":\"d3a7e232-15f2-47a9-a065-9480c81dc57e\"},{\"content\":{\"connectorIds\":[\"Out1\"],\"side\":\"RIGHT\"},\"type\":\"ConnectorPlacement.EquallySpacedRectSide\",\"uuid\":\"e118f150-fee7-4aeb-941e-53c3f02c6791\"},{\"content\":{\"connectorIds\":[\"Out2\"],\"side\":\"TOP\"},\"type\":\"ConnectorPlacement.EquallySpacedRectSide\",\"uuid\":\"6d9038ab-faad-455b-a9c5-8fe0bbf34e51\"},{\"content\":{\"connectorIds\":[\"In2\"],\"side\":\"BOTTOM\"},\"type\":\"ConnectorPlacement.EquallySpacedRectSide\",\"uuid\":\"d09c8d4f-08f3-4c52-88a6-8c6db517fc7a\"}]},\"type\":\"ConnectorPlacement.EquallySpacedConnector\",\"uuid\":\"5bc947ce-f1cd-4957-9186-40c14c78de7d\"}],\"packageUris\":[\"http://schema.mathworks.com/mf0/Connector/R2020b\"],\"version\":\"1.0\"}"
  Half Adder2 : Subsystem
      settings: PortSchema="{\"entries\":[{\"content\":{\"sides\":[{\"content\":{\"connectorIds\":[\"In1\"]},\"type\":\"ConnectorPlacement.EquallySpacedRectSide\",\"uuid\":\"d3a7e232-15f2-47a9-a065-9480c81dc57e\"},{\"content\":{\"connectorIds\":[\"Out1\"],\"side\":\"RIGHT\"},\"type\":\"ConnectorPlacement.EquallySpacedRectSide\",\"uuid\":\"e118f150-fee7-4aeb-941e-53c3f02c6791\"},{\"content\":{\"connectorIds\":[\"Out2\"],\"side\":\"TOP\"},\"type\":\"ConnectorPlacement.EquallySpacedRectSide\",\"uuid\":\"6d9038ab-faad-455b-a9c5-8fe0bbf34e51\"},{\"content\":{\"connectorIds\":[\"In2\"],\"side\":\"BOTTOM\"},\"type\":\"ConnectorPlacement.EquallySpacedRectSide\",\"uuid\":\"d09c8d4f-08f3-4c52-88a6-8c6db517fc7a\"}]},\"type\":\"ConnectorPlacement.EquallySpacedConnector\",\"uuid\":\"5bc947ce-f1cd-4957-9186-40c14c78de7d\"}],\"packageUris\":[\"http://schema.mathworks.com/mf0/Connector/R2020b\"],\"version\":\"1.0\"}"
  Half Adder3 : Subsystem
      settings: PortSchema="{\"entries\":[{\"content\":{\"sides\":[{\"content\":{\"connectorIds\":[\"In1\"]},\"type\":\"ConnectorPlacement.EquallySpacedRectSide\",\"uuid\":\"d3a7e232-15f2-47a9-a065-9480c81dc57e\"},{\"content\":{\"connectorIds\":[\"Out1\"],\"side\":\"RIGHT\"},\"type\":\"ConnectorPlacement.EquallySpacedRectSide\",\"uuid\":\"e118f150-fee7-4aeb-941e-53c3f02c6791\"},{\"content\":{\"connectorIds\":[\"Out2\"],\"side\":\"TOP\"},\"type\":\"ConnectorPlacement.EquallySpacedRectSide\",\"uuid\":\"6d9038ab-faad-455b-a9c5-8fe0bbf34e51\"},{\"content\":{\"connectorIds\":[\"In2\"],\"side\":\"BOTTOM\"},\"type\":\"ConnectorPlacement.EquallySpacedRectSide\",\"uuid\":\"d09c8d4f-08f3-4c52-88a6-8c6db517fc7a\"}]},\"type\":\"ConnectorPlacement.EquallySpacedConnector\",\"uuid\":\"5bc947ce-f1cd-4957-9186-40c14c78de7d\"}],\"packageUris\":[\"http://schema.mathworks.com/mf0/Connector/R2020b\"],\"version\":\"1.0\"}"
  Half Adder4 : Subsystem
      settings: PortSchema="{\"entries\":[{\"content\":{\"sides\":[{\"content\":{\"connectorIds\":[\"In1\"]},\"type\":\"ConnectorPlacement.EquallySpacedRectSide\",\"uuid\":\"d3a7e232-15f2-47a9-a065-9480c81dc57e\"},{\"content\":{\"connectorIds\":[\"Out1\"],\"side\":\"RIGHT\"},\"type\":\"ConnectorPlacement.EquallySpacedRectSide\",\"uuid\":\"e118f150-fee7-4aeb-941e-53c3f02c6791\"},{\"content\":{\"connectorIds\":[\"Out2\"],\"side\":\"TOP\"},\"type\":\"ConnectorPlacement.EquallySpacedRectSide\",\"uuid\":\"6d9038ab-faad-455b-a9c5-8fe0bbf34e51\"},{\"content\":{\"connectorIds\":[\"In2\"],\"side\":\"BOTTOM\"},\"type\":\"ConnectorPlacement.EquallySpacedRectSide\",\"uuid\":\"d09c8d4f-08f3-4c52-88a6-8c6db517fc7a\"}]},\"type\":\"ConnectorPlacement.EquallySpacedConnector\",\"uuid\":\"5bc947ce-f1cd-4957-9186-40c14c78de7d\"}],\"packageUris\":[\"http://schema.mathworks.com/mf0/Connector/R2020b\"],\"version\":\"1.0\"}"
  Half Adder5 : Subsystem
      settings: PortSchema="{\"entries\":[{\"content\":{\"sides\":[{\"content\":{\"connectorIds\":[\"In1\"]},\"type\":\"ConnectorPlacement.EquallySpacedRectSide\",\"uuid\":\"d3a7e232-15f2-47a9-a065-9480c81dc57e\"},{\"content\":{\"connectorIds\":[\"Out1\"],\"side\":\"RIGHT\"},\"type\":\"ConnectorPlacement.EquallySpacedRectSide\",\"uuid\":\"e118f150-fee7-4aeb-941e-53c3f02c6791\"},{\"content\":{\"connectorIds\":[\"Out2\"],\"side\":\"TOP\"},\"type\":\"ConnectorPlacement.EquallySpacedRectSide\",\"uuid\":\"6d9038ab-faad-455b-a9c5-8fe0bbf34e51\"},{\"content\":{\"connectorIds\":[\"In2\"],\"side\":\"BOTTOM\"},\"type\":\"ConnectorPlacement.EquallySpacedRectSide\",\"uuid\":\"d09c8d4f-08f3-4c52-88a6-8c6db517fc7a\"}]},\"type\":\"ConnectorPlacement.EquallySpacedConnector\",\"uuid\":\"5bc947ce-f1cd-4957-9186-40c14c78de7d\"}],\"packageUris\":[\"http://schema.mathworks.com/mf0/Connector/R2020b\"],\"version\":\"1.0\"}"
  Half Adder6 : Subsystem
      settings: PortSchema="{\"entries\":[{\"content\":{\"sides\":[{\"content\":{\"connectorIds\":[\"In1\"]},\"type\":\"ConnectorPlacement.EquallySpacedRectSide\",\"uuid\":\"d3a7e232-15f2-47a9-a065-9480c81dc57e\"},{\"content\":{\"connectorIds\":[\"Out1\"],\"side\":\"RIGHT\"},\"type\":\"ConnectorPlacement.EquallySpacedRectSide\",\"uuid\":\"e118f150-fee7-4aeb-941e-53c3f02c6791\"},{\"content\":{\"side\":\"TOP\"},\"type\":\"ConnectorPlacement.EquallySpacedRectSide\",\"uuid\":\"6d9038ab-faad-455b-a9c5-8fe0bbf34e51\"},{\"content\":{\"connectorIds\":[\"In2\"],\"side\":\"BOTTOM\"},\"type\":\"ConnectorPlacement.EquallySpacedRectSide\",\"uuid\":\"d09c8d4f-08f3-4c52-88a6-8c6db517fc7a\"}]},\"type\":\"ConnectorPlacement.EquallySpacedConnector\",\"uuid\":\"5bc947ce-f1cd-4957-9186-40c14c78de7d\"}],\"packageUris\":[\"http://schema.mathworks.com/mf0/Connector/R2020b\"],\"version\":\"1.0\"}"
  Half Adder7 : Subsystem
      settings: PortSchema="{\"entries\":[{\"content\":{\"sides\":[{\"content\":{\"connectorIds\":[\"In1\"]},\"type\":\"ConnectorPlacement.EquallySpacedRectSide\",\"uuid\":\"d3a7e232-15f2-47a9-a065-9480c81dc57e\"},{\"content\":{\"connectorIds\":[\"Out1\"],\"side\":\"RIGHT\"},\"type\":\"ConnectorPlacement.EquallySpacedRectSide\",\"uuid\":\"e118f150-fee7-4aeb-941e-53c3f02c6791\"},{\"content\":{\"connectorIds\":[\"Out2\"],\"side\":\"TOP\"},\"type\":\"ConnectorPlacement.EquallySpacedRectSide\",\"uuid\":\"6d9038ab-faad-455b-a9c5-8fe0bbf34e51\"},{\"content\":{\"connectorIds\":[\"In2\"],\"side\":\"BOTTOM\"},\"type\":\"ConnectorPlacement.EquallySpacedRectSide\",\"uuid\":\"d09c8d4f-08f3-4c52-88a6-8c6db517fc7a\"}]},\"type\":\"ConnectorPlacement.EquallySpacedConnector\",\"uuid\":\"5bc947ce-f1cd-4957-9186-40c14c78de7d\"}],\"packageUris\":[\"http://schema.mathworks.com/mf0/Connector/R2020b\"],\"version\":\"1.0\"}"
  Mux1 : Mux  Inputs=8
  Mux2 : Mux  Inputs=8
  NOT : Logic  Operator=NOT  IconShape=distinctive  AllPortsSameDT=off  OutDataTypeStr=boolean
  TC : Outport
  wires:
  Mux1/1 -> Delay One Step/1
  TC_RST/1 -> NOT/1
  Delay One Step/1 -> Demux/1
  Demux/4 -> D Flip-Flop4/1
  Demux/3 -> D Flip-Flop2/1
  Demux/2 -> D Flip-Flop3/1
  Demux/1 -> D Flip-Flop1/1
  Demux/8 -> D Flip-Flop7/1
  Demux/7 -> D Flip-Flop5/1
  Demux/6 -> D Flip-Flop6/1
  Demux/5 -> D Flip-Flop11/1
  INC/1 -> D Flip-Flop2/2, D Flip-Flop3/2, D Flip-Flop1/2, D Flip-Flop4/2, D Flip-Flop11/2, D Flip-Flop6/2, D Flip-Flop5/2, D Flip-Flop7/2
  Constant/1 -> Half Adder7/2("B ")
  Half Adder5/2(Carry) -> Half Adder6/2("B ")
  Half Adder/2(Carry) -> Half Adder1/2("B ")
  Half Adder4/1(Sum) -> Mux1/3
  Half Adder6/1(Sum) -> Mux1/1
  Half Adder5/1(Sum) -> Mux1/2
  Half Adder1/1(Sum) -> Mux1/6
  Half Adder/1(Sum) -> Mux1/7
  Half Adder2/1(Sum) -> Mux1/5
  Half Adder2/2(Carry) -> Half Adder3/2("B ")
  Half Adder3/1(Sum) -> Mux1/4
  Half Adder4/2(Carry) -> Half Adder5/2("B ")
  Half Adder3/2(Carry) -> Half Adder4/2("B ")
  Half Adder1/2(Carry) -> Half Adder2/2("B ")
  Half Adder7/1(Sum) -> Mux1/8
  Half Adder7/2(Carry) -> Half Adder/2("B ")
  D Flip-Flop1/1 -> Mux2/1, Half Adder6/1(A)  "D1"
  D Flip-Flop3/1 -> Mux2/2, Half Adder5/1(A)  "D3"
  D Flip-Flop2/1 -> Mux2/3, Half Adder4/1(A)  "D4"
  D Flip-Flop4/1 -> Mux2/4, Half Adder3/1(A)  "D2"
  D Flip-Flop11/1 -> Mux2/5, Half Adder2/1(A)  "D1"
  D Flip-Flop6/1 -> Mux2/6, Half Adder1/1(A)  "D3"
  D Flip-Flop5/1 -> Mux2/7, Half Adder/1(A)  "D4"
  D Flip-Flop7/1 -> Mux2/8, Half Adder7/1(A)  "D2"
  Mux2/1 -> TC/1
  NOT/1 -> D Flip-Flop2/3, D Flip-Flop1/3, D Flip-Flop3/3, D Flip-Flop4/3, D Flip-Flop11/3, D Flip-Flop6/3, D Flip-Flop5/3, D Flip-Flop7/3

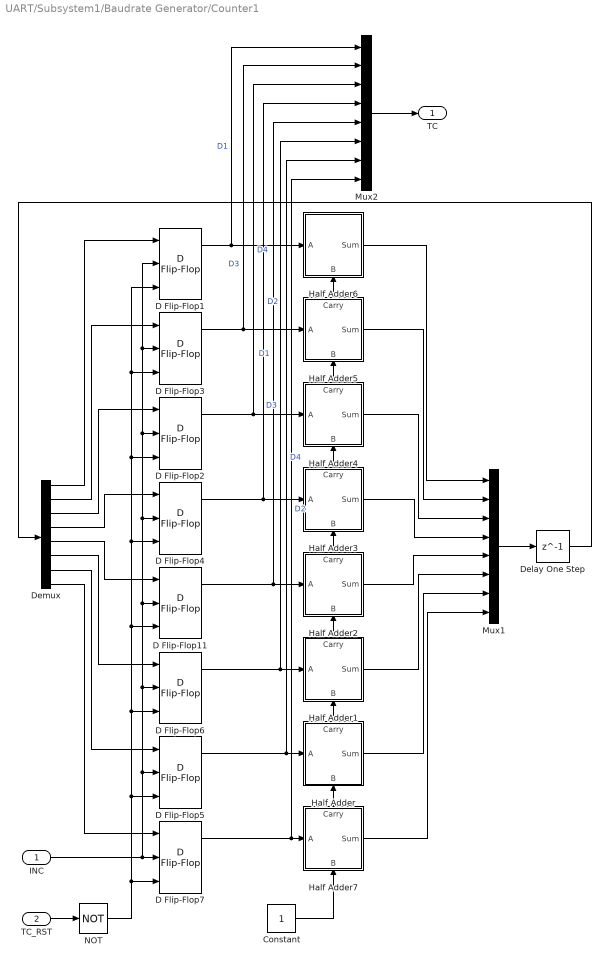
== system UART/Subsystem1/Baudrate Generator/Counter1 ==
  INC : Inport
  TC_RST : Inport  Port=2
  Constant : Constant
  D Flip-Flop{1..7,11} (8 alike) : simulink_extras/Flip Flops/D Flip-Flop
  Delay One Step : Delay  DelayLength=1
  Demux : Demux  Outputs=8
  Half Adder : Subsystem
      settings: PortSchema="{\"entries\":[{\"content\":{\"sides\":[{\"content\":{\"connectorIds\":[\"In1\"]},\"type\":\"ConnectorPlacement.EquallySpacedRectSide\",\"uuid\":\"d3a7e232-15f2-47a9-a065-9480c81dc57e\"},{\"content\":{\"connectorIds\":[\"Out1\"],\"side\":\"RIGHT\"},\"type\":\"ConnectorPlacement.EquallySpacedRectSide\",\"uuid\":\"e118f150-fee7-4aeb-941e-53c3f02c6791\"},{\"content\":{\"connectorIds\":[\"Out2\"],\"side\":\"TOP\"},\"type\":\"ConnectorPlacement.EquallySpacedRectSide\",\"uuid\":\"6d9038ab-faad-455b-a9c5-8fe0bbf34e51\"},{\"content\":{\"connectorIds\":[\"In2\"],\"side\":\"BOTTOM\"},\"type\":\"ConnectorPlacement.EquallySpacedRectSide\",\"uuid\":\"d09c8d4f-08f3-4c52-88a6-8c6db517fc7a\"}]},\"type\":\"ConnectorPlacement.EquallySpacedConnector\",\"uuid\":\"5bc947ce-f1cd-4957-9186-40c14c78de7d\"}],\"packageUris\":[\"http://schema.mathworks.com/mf0/Connector/R2020b\"],\"version\":\"1.0\"}"
  Half Adder1 : Subsystem
      settings: PortSchema="{\"entries\":[{\"content\":{\"sides\":[{\"content\":{\"connectorIds\":[\"In1\"]},\"type\":\"ConnectorPlacement.EquallySpacedRectSide\",\"uuid\":\"d3a7e232-15f2-47a9-a065-9480c81dc57e\"},{\"content\":{\"connectorIds\":[\"Out1\"],\"side\":\"RIGHT\"},\"type\":\"ConnectorPlacement.EquallySpacedRectSide\",\"uuid\":\"e118f150-fee7-4aeb-941e-53c3f02c6791\"},{\"content\":{\"connectorIds\":[\"Out2\"],\"side\":\"TOP\"},\"type\":\"ConnectorPlacement.EquallySpacedRectSide\",\"uuid\":\"6d9038ab-faad-455b-a9c5-8fe0bbf34e51\"},{\"content\":{\"connectorIds\":[\"In2\"],\"side\":\"BOTTOM\"},\"type\":\"ConnectorPlacement.EquallySpacedRectSide\",\"uuid\":\"d09c8d4f-08f3-4c52-88a6-8c6db517fc7a\"}]},\"type\":\"ConnectorPlacement.EquallySpacedConnector\",\"uuid\":\"5bc947ce-f1cd-4957-9186-40c14c78de7d\"}],\"packageUris\":[\"http://schema.mathworks.com/mf0/Connector/R2020b\"],\"version\":\"1.0\"}"
  Half Adder2 : Subsystem
      settings: PortSchema="{\"entries\":[{\"content\":{\"sides\":[{\"content\":{\"connectorIds\":[\"In1\"]},\"type\":\"ConnectorPlacement.EquallySpacedRectSide\",\"uuid\":\"d3a7e232-15f2-47a9-a065-9480c81dc57e\"},{\"content\":{\"connectorIds\":[\"Out1\"],\"side\":\"RIGHT\"},\"type\":\"ConnectorPlacement.EquallySpacedRectSide\",\"uuid\":\"e118f150-fee7-4aeb-941e-53c3f02c6791\"},{\"content\":{\"connectorIds\":[\"Out2\"],\"side\":\"TOP\"},\"type\":\"ConnectorPlacement.EquallySpacedRectSide\",\"uuid\":\"6d9038ab-faad-455b-a9c5-8fe0bbf34e51\"},{\"content\":{\"connectorIds\":[\"In2\"],\"side\":\"BOTTOM\"},\"type\":\"ConnectorPlacement.EquallySpacedRectSide\",\"uuid\":\"d09c8d4f-08f3-4c52-88a6-8c6db517fc7a\"}]},\"type\":\"ConnectorPlacement.EquallySpacedConnector\",\"uuid\":\"5bc947ce-f1cd-4957-9186-40c14c78de7d\"}],\"packageUris\":[\"http://schema.mathworks.com/mf0/Connector/R2020b\"],\"version\":\"1.0\"}"
  Half Adder3 : Subsystem
      settings: PortSchema="{\"entries\":[{\"content\":{\"sides\":[{\"content\":{\"connectorIds\":[\"In1\"]},\"type\":\"ConnectorPlacement.EquallySpacedRectSide\",\"uuid\":\"d3a7e232-15f2-47a9-a065-9480c81dc57e\"},{\"content\":{\"connectorIds\":[\"Out1\"],\"side\":\"RIGHT\"},\"type\":\"ConnectorPlacement.EquallySpacedRectSide\",\"uuid\":\"e118f150-fee7-4aeb-941e-53c3f02c6791\"},{\"content\":{\"connectorIds\":[\"Out2\"],\"side\":\"TOP\"},\"type\":\"ConnectorPlacement.EquallySpacedRectSide\",\"uuid\":\"6d9038ab-faad-455b-a9c5-8fe0bbf34e51\"},{\"content\":{\"connectorIds\":[\"In2\"],\"side\":\"BOTTOM\"},\"type\":\"ConnectorPlacement.EquallySpacedRectSide\",\"uuid\":\"d09c8d4f-08f3-4c52-88a6-8c6db517fc7a\"}]},\"type\":\"ConnectorPlacement.EquallySpacedConnector\",\"uuid\":\"5bc947ce-f1cd-4957-9186-40c14c78de7d\"}],\"packageUris\":[\"http://schema.mathworks.com/mf0/Connector/R2020b\"],\"version\":\"1.0\"}"
  Half Adder4 : Subsystem
      settings: PortSchema="{\"entries\":[{\"content\":{\"sides\":[{\"content\":{\"connectorIds\":[\"In1\"]},\"type\":\"ConnectorPlacement.EquallySpacedRectSide\",\"uuid\":\"d3a7e232-15f2-47a9-a065-9480c81dc57e\"},{\"content\":{\"connectorIds\":[\"Out1\"],\"side\":\"RIGHT\"},\"type\":\"ConnectorPlacement.EquallySpacedRectSide\",\"uuid\":\"e118f150-fee7-4aeb-941e-53c3f02c6791\"},{\"content\":{\"connectorIds\":[\"Out2\"],\"side\":\"TOP\"},\"type\":\"ConnectorPlacement.EquallySpacedRectSide\",\"uuid\":\"6d9038ab-faad-455b-a9c5-8fe0bbf34e51\"},{\"content\":{\"connectorIds\":[\"In2\"],\"side\":\"BOTTOM\"},\"type\":\"ConnectorPlacement.EquallySpacedRectSide\",\"uuid\":\"d09c8d4f-08f3-4c52-88a6-8c6db517fc7a\"}]},\"type\":\"ConnectorPlacement.EquallySpacedConnector\",\"uuid\":\"5bc947ce-f1cd-4957-9186-40c14c78de7d\"}],\"packageUris\":[\"http://schema.mathworks.com/mf0/Connector/R2020b\"],\"version\":\"1.0\"}"
  Half Adder5 : Subsystem
      settings: PortSchema="{\"entries\":[{\"content\":{\"sides\":[{\"content\":{\"connectorIds\":[\"In1\"]},\"type\":\"ConnectorPlacement.EquallySpacedRectSide\",\"uuid\":\"d3a7e232-15f2-47a9-a065-9480c81dc57e\"},{\"content\":{\"connectorIds\":[\"Out1\"],\"side\":\"RIGHT\"},\"type\":\"ConnectorPlacement.EquallySpacedRectSide\",\"uuid\":\"e118f150-fee7-4aeb-941e-53c3f02c6791\"},{\"content\":{\"connectorIds\":[\"Out2\"],\"side\":\"TOP\"},\"type\":\"ConnectorPlacement.EquallySpacedRectSide\",\"uuid\":\"6d9038ab-faad-455b-a9c5-8fe0bbf34e51\"},{\"content\":{\"connectorIds\":[\"In2\"],\"side\":\"BOTTOM\"},\"type\":\"ConnectorPlacement.EquallySpacedRectSide\",\"uuid\":\"d09c8d4f-08f3-4c52-88a6-8c6db517fc7a\"}]},\"type\":\"ConnectorPlacement.EquallySpacedConnector\",\"uuid\":\"5bc947ce-f1cd-4957-9186-40c14c78de7d\"}],\"packageUris\":[\"http://schema.mathworks.com/mf0/Connector/R2020b\"],\"version\":\"1.0\"}"
  Half Adder6 : Subsystem
      settings: PortSchema="{\"entries\":[{\"content\":{\"sides\":[{\"content\":{\"connectorIds\":[\"In1\"]},\"type\":\"ConnectorPlacement.EquallySpacedRectSide\",\"uuid\":\"d3a7e232-15f2-47a9-a065-9480c81dc57e\"},{\"content\":{\"connectorIds\":[\"Out1\"],\"side\":\"RIGHT\"},\"type\":\"ConnectorPlacement.EquallySpacedRectSide\",\"uuid\":\"e118f150-fee7-4aeb-941e-53c3f02c6791\"},{\"content\":{\"side\":\"TOP\"},\"type\":\"ConnectorPlacement.EquallySpacedRectSide\",\"uuid\":\"6d9038ab-faad-455b-a9c5-8fe0bbf34e51\"},{\"content\":{\"connectorIds\":[\"In2\"],\"side\":\"BOTTOM\"},\"type\":\"ConnectorPlacement.EquallySpacedRectSide\",\"uuid\":\"d09c8d4f-08f3-4c52-88a6-8c6db517fc7a\"}]},\"type\":\"ConnectorPlacement.EquallySpacedConnector\",\"uuid\":\"5bc947ce-f1cd-4957-9186-40c14c78de7d\"}],\"packageUris\":[\"http://schema.mathworks.com/mf0/Connector/R2020b\"],\"version\":\"1.0\"}"
  Half Adder7 : Subsystem
      settings: PortSchema="{\"entries\":[{\"content\":{\"sides\":[{\"content\":{\"connectorIds\":[\"In1\"]},\"type\":\"ConnectorPlacement.EquallySpacedRectSide\",\"uuid\":\"d3a7e232-15f2-47a9-a065-9480c81dc57e\"},{\"content\":{\"connectorIds\":[\"Out1\"],\"side\":\"RIGHT\"},\"type\":\"ConnectorPlacement.EquallySpacedRectSide\",\"uuid\":\"e118f150-fee7-4aeb-941e-53c3f02c6791\"},{\"content\":{\"connectorIds\":[\"Out2\"],\"side\":\"TOP\"},\"type\":\"ConnectorPlacement.EquallySpacedRectSide\",\"uuid\":\"6d9038ab-faad-455b-a9c5-8fe0bbf34e51\"},{\"content\":{\"connectorIds\":[\"In2\"],\"side\":\"BOTTOM\"},\"type\":\"ConnectorPlacement.EquallySpacedRectSide\",\"uuid\":\"d09c8d4f-08f3-4c52-88a6-8c6db517fc7a\"}]},\"type\":\"ConnectorPlacement.EquallySpacedConnector\",\"uuid\":\"5bc947ce-f1cd-4957-9186-40c14c78de7d\"}],\"packageUris\":[\"http://schema.mathworks.com/mf0/Connector/R2020b\"],\"version\":\"1.0\"}"
  Mux1 : Mux  Inputs=8
  Mux2 : Mux  Inputs=8
  NOT : Logic  Operator=NOT  IconShape=distinctive  AllPortsSameDT=off  OutDataTypeStr=boolean
  TC : Outport
  wires:
  Mux1/1 -> Delay One Step/1
  TC_RST/1 -> NOT/1
  Delay One Step/1 -> Demux/1
  Demux/4 -> D Flip-Flop4/1
  Demux/3 -> D Flip-Flop2/1
  Demux/2 -> D Flip-Flop3/1
  Demux/1 -> D Flip-Flop1/1
  Demux/8 -> D Flip-Flop7/1
  Demux/7 -> D Flip-Flop5/1
  Demux/6 -> D Flip-Flop6/1
  Demux/5 -> D Flip-Flop11/1
  INC/1 -> D Flip-Flop2/2, D Flip-Flop3/2, D Flip-Flop1/2, D Flip-Flop4/2, D Flip-Flop11/2, D Flip-Flop6/2, D Flip-Flop5/2, D Flip-Flop7/2
  Constant/1 -> Half Adder7/2("B ")
  Half Adder5/2(Carry) -> Half Adder6/2("B ")
  Half Adder/2(Carry) -> Half Adder1/2("B ")
  Half Adder4/1(Sum) -> Mux1/3
  Half Adder6/1(Sum) -> Mux1/1
  Half Adder5/1(Sum) -> Mux1/2
  Half Adder1/1(Sum) -> Mux1/6
  Half Adder/1(Sum) -> Mux1/7
  Half Adder2/1(Sum) -> Mux1/5
  Half Adder2/2(Carry) -> Half Adder3/2("B ")
  Half Adder3/1(Sum) -> Mux1/4
  Half Adder4/2(Carry) -> Half Adder5/2("B ")
  Half Adder3/2(Carry) -> Half Adder4/2("B ")
  Half Adder1/2(Carry) -> Half Adder2/2("B ")
  Half Adder7/1(Sum) -> Mux1/8
  Half Adder7/2(Carry) -> Half Adder/2("B ")
  D Flip-Flop1/1 -> Mux2/1, Half Adder6/1(A)  "D1"
  D Flip-Flop3/1 -> Mux2/2, Half Adder5/1(A)  "D3"
  D Flip-Flop2/1 -> Mux2/3, Half Adder4/1(A)  "D4"
  D Flip-Flop4/1 -> Mux2/4, Half Adder3/1(A)  "D2"
  D Flip-Flop11/1 -> Mux2/5, Half Adder2/1(A)  "D1"
  D Flip-Flop6/1 -> Mux2/6, Half Adder1/1(A)  "D3"
  D Flip-Flop5/1 -> Mux2/7, Half Adder/1(A)  "D4"
  D Flip-Flop7/1 -> Mux2/8, Half Adder7/1(A)  "D2"
  Mux2/1 -> TC/1
  NOT/1 -> D Flip-Flop2/3, D Flip-Flop1/3, D Flip-Flop3/3, D Flip-Flop4/3, D Flip-Flop11/3, D Flip-Flop6/3, D Flip-Flop5/3, D Flip-Flop7/3

== system UART/Subsystem1/Baudrate Generator/Prescaler_Controller1 ==
  "CLR " : Inport
  TReg : Inport  Port=2
  Enable : Inport  Port=3
  StoreTReg : Inport  Port=4
  CLK : Inport  Port=5
  TC : Inport  Port=6
  AND{,1..3} (4 alike) : Logic  IconShape=distinctive  AllPortsSameDT=off  OutDataTypeStr=boolean
  Delay One Step : Delay  DelayLength=1
  Demux : Demux  Outputs=8
  NOR : Logic  Operator=NOR  Inputs=8  IconShape=distinctive  AllPortsSameDT=off  OutDataTypeStr=boolean
  NOT : Logic  Operator=NOT  IconShape=distinctive  AllPortsSameDT=off  OutDataTypeStr=boolean
  NOT1 : Logic  Operator=NOT  IconShape=distinctive  AllPortsSameDT=off  OutDataTypeStr=boolean
  OR : Logic  Operator=OR  Inputs=3  IconShape=distinctive  AllPortsSameDT=off  OutDataTypeStr=boolean
  S-R Flip-Flop : simulink_extras/Flip Flops/S-R Flip-Flop  initial_condition=0
  Scope : Scope
      settings: ActiveDisplayYMinimum=-1  ActiveDisplayYMaximum=1  DataLoggingVariableName=ScopeData2
  XOR : Logic  Operator=XOR  IconShape=distinctive  AllPortsSameDT=off  OutDataTypeStr=boolean
  CLK_Next : Outport
  INC : Outport  Port=2
  TC_RST : Outport  Port=3
  wires:
  TReg/1 -> XOR/1
  Demux/1 -> NOR/1
  TC/1 -> XOR/2
  XOR/1 -> Demux/1
  Demux/2 -> NOR/2
  Demux/3 -> NOR/3
  Demux/4 -> NOR/4
  Demux/5 -> NOR/5
  Demux/6 -> NOR/6
  Demux/7 -> NOR/7
  Demux/8 -> NOR/8
  "CLR "/1 -> OR/3
  NOR/1 -> NOT/1, AND1/1
  Enable/1 -> AND1/2, AND/1
  OR/1 -> Delay One Step/1
  StoreTReg/1 -> OR/1
  AND/1 -> INC/1
  Delay One Step/1 -> AND3/1, TC_RST/1
  AND1/1 -> S-R Flip-Flop/1
  S-R Flip-Flop/1 -> AND2/2
  NOT/1 -> AND2/1
  AND2/1 -> OR/2, Scope/1, CLK_Next/1
  CLK/1 -> NOT1/1, AND/2
  AND3/1 -> S-R Flip-Flop/2
  NOT1/1 -> AND3/2

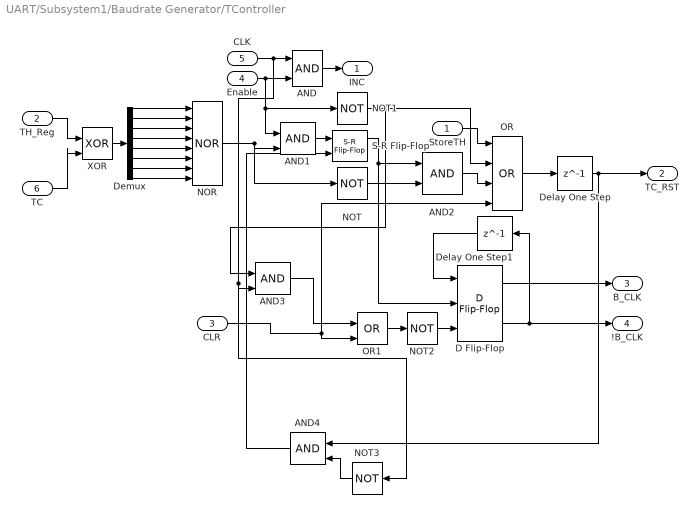
== system UART/Subsystem1/Baudrate Generator/TController ==
  StoreTH : Inport
  TH_Reg : Inport  Port=2
  "CLR " : Inport  Port=3
  Enable : Inport  Port=4
  CLK : Inport  Port=5
  TC : Inport  Port=6
  AND{,1..4} (5 alike) : Logic  IconShape=distinctive  AllPortsSameDT=off  OutDataTypeStr=boolean
  D Flip-Flop : simulink_extras/Flip Flops/D Flip-Flop
  Delay One Step : Delay  DelayLength=1
  Delay One Step1 : Delay  DelayLength=1
  Demux : Demux  Outputs=8
  NOR : Logic  Operator=NOR  Inputs=8  IconShape=distinctive  AllPortsSameDT=off  OutDataTypeStr=boolean
  NOT{,1..3} (4 alike) : Logic  Operator=NOT  IconShape=distinctive  AllPortsSameDT=off  OutDataTypeStr=boolean
  OR : Logic  Operator=OR  Inputs=4  IconShape=distinctive  AllPortsSameDT=off  OutDataTypeStr=boolean
  OR1 : Logic  Operator=OR  IconShape=distinctive  AllPortsSameDT=off  OutDataTypeStr=boolean
  S-R Flip-Flop : simulink_extras/Flip Flops/S-R Flip-Flop  initial_condition=0
  XOR : Logic  Operator=XOR  IconShape=distinctive  AllPortsSameDT=off  OutDataTypeStr=boolean
  INC : Outport
  TC_RST : Outport  Port=2
  B_CLK : Outport  Port=3
  !B_CLK : Outport  Port=4
  wires:
  TH_Reg/1 -> XOR/1
  Demux/1 -> NOR/1
  TC/1 -> XOR/2
  XOR/1 -> Demux/1
  Demux/2 -> NOR/2
  Demux/3 -> NOR/3
  Demux/4 -> NOR/4
  Demux/5 -> NOR/5
  Demux/6 -> NOR/6
  Demux/7 -> NOR/7
  Demux/8 -> NOR/8
  AND1/1 -> S-R Flip-Flop/1
  Enable/1 -> NOT1/1, AND1/1, AND/2
  AND2/1 -> OR/3
  OR/1 -> Delay One Step/1
  Delay One Step/1 -> AND4/1, TC_RST/1
  CLK/1 -> NOT3/1, AND3/2, AND/1
  S-R Flip-Flop/1 -> D Flip-Flop/2, AND2/1
  D Flip-Flop/2 -> Delay One Step1/1, !B_CLK/1
  Delay One Step1/1 -> D Flip-Flop/1
  StoreTH/1 -> OR/1
  D Flip-Flop/1 -> B_CLK/1
  NOR/1 -> NOT/1, AND1/2
  AND/1 -> INC/1
  "CLR "/1 -> OR/4, OR1/2
  NOT2/1 -> D Flip-Flop/3
  NOT/1 -> AND2/2
  NOT1/1 -> AND3/1, OR/2
  OR1/1 -> NOT2/1
  AND3/1 -> OR1/1
  NOT3/1 -> AND4/2
  AND4/1 -> S-R Flip-Flop/2

== system UART/Subsystem1/PISO/Subsystem1 ==
  Data : Inport
  Clock : Inport  Port=2
  CLR : Inport  Port=3
  Store : Inport  Port=4
  AND : Logic  IconShape=distinctive  AllPortsSameDT=off  OutDataTypeStr=boolean
  AND1 : Logic  IconShape=distinctive  AllPortsSameDT=off  OutDataTypeStr=boolean
  D Flip-Flop : simulink_extras/Flip Flops/D Flip-Flop
  NOT : Logic  Operator=NOT  IconShape=distinctive  AllPortsSameDT=off  OutDataTypeStr=boolean
  NOT1 : Logic  Operator=NOT  IconShape=distinctive  AllPortsSameDT=off  OutDataTypeStr=boolean
  OR : Logic  Operator=OR  IconShape=distinctive  AllPortsSameDT=off  OutDataTypeStr=boolean
  Q : Outport
  !Q : Outport  Port=2
  wires:
  AND1/1 -> OR/2
  AND/1 -> OR/1
  D Flip-Flop/1 -> Q/1, AND1/2
  NOT/1 -> AND1/1
  Store/1 -> AND/2, NOT/1
  Clock/1 -> D Flip-Flop/2
  Data/1 -> AND/1
  OR/1 -> D Flip-Flop/1
  D Flip-Flop/2 -> !Q/1
  CLR/1 -> NOT1/1
  NOT1/1 -> D Flip-Flop/3
